simulink model "Assignment_1"  (R2020b)
settings: Solver=VariableStepAuto  StartTime=0.0  StopTime=100  RelTol=1e-3
values from neighbouring files (symbols this model uses):
  b = 50    [Values.m]
  K1 = 50    [Values.m]
  K12 = 120    [Values.m]
  M1 = 100    [Values.m]
  M2 = 30    [Values.m]
settings Model: Creator=Shantam Garg  LastModifiedBy=Shantam Garg

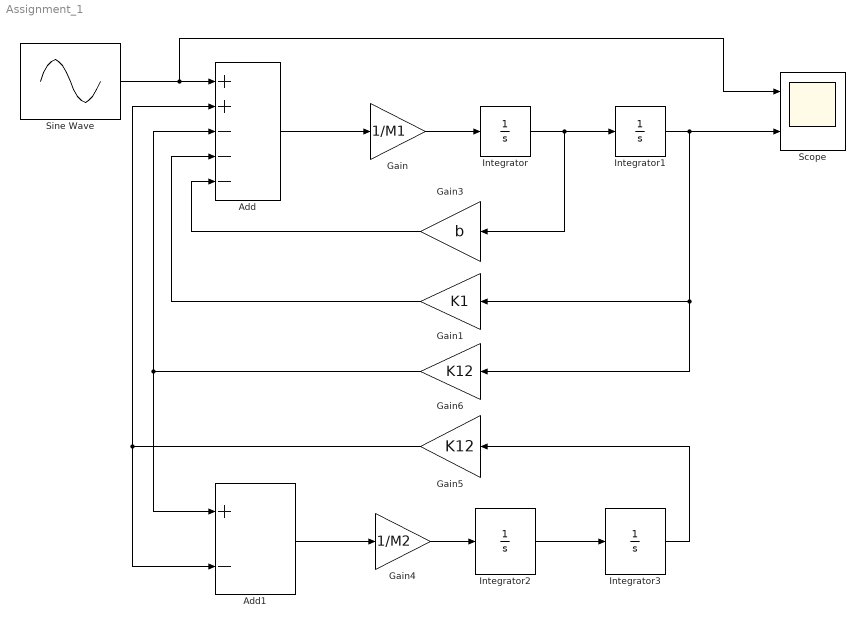
== system Assignment_1 ==
  Add : Sum  Inputs=++---
  Add1 : Sum  Inputs=+-
  Gain : Gain  Gain=1/M1
  Gain1 : Gain  Gain=K1
  Gain3 : Gain  Gain=b
  Gain4 : Gain  Gain=1/M2
  Gain5 : Gain  Gain=K12
  Gain6 : Gain  Gain=K12
  Integrator{,1..3} (4 alike) : Integrator
  Scope : Scope  NumInputPorts=2
  Sine Wave : Sin  Amplitude=2  Frequency=10  SampleTime=0
  wires:
  Add/1 -> Gain/1
  Gain/1 -> Integrator/1
  Integrator/1 -> Gain3/1, Integrator1/1
  Gain3/1 -> Add/5
  Add1/1 -> Gain4/1
  Gain4/1 -> Integrator2/1
  Integrator2/1 -> Integrator3/1
  Gain1/1 -> Add/4
  Sine Wave/1 -> Scope/1, Add/1
  Gain5/1 -> Add/2, Add1/2
  Integrator3/1 -> Gain5/1
  Gain6/1 -> Add/3, Add1/1
  Integrator1/1 -> Gain6/1, Gain1/1, Scope/2
